simulink model "rolling_mill"  (R2017b)
settings: Solver=ode14x  StartTime=0.0  StopTime=500  FixedStep=0.01  RelTol=1e-3  EnableMultiTasking=on
PreLoadFcn:
  | load rolling_mill
  | preload
values from neighbouring files (symbols this model uses):
  gx = 1e-6    (= 1e-06)    [milldemo.m]
  gxy = 0.1    [milldemo.m]
  gy = 0.5e-6    (= 5e-07)    [milldemo.m]
  gyx = 0.4    [milldemo.m]
libraries: cstblocks x8, simulink x4
settings Model: Creator=The MathWorks, Inc.  LastModifiedBy=matlab
settings DataIOCC: LimitDataPoints=on  SaveFormat=Array
settings OptimizationCC: BlockReduction=off  BooleanDataType=off  InitFltsAndDblsToZero=on
settings DebuggingCC: SaveWithParameterizedLinksMsg=none  UnderspecifiedInitializationDetection=Classic  MergeDetectMultiDrivingBlocksExec=none  SignalResolutionControl=TryResolveAllWithWarning  MultiTaskDSMMsg=warning  MultiTaskCondExecSysMsg=none  FcnCallInpInsideContextMsg=warning  StateNameClashWarn=warning  StrictBusMsg=None  SFUnexpectedBacktrackingDiag=warning  SFNoUnconditionalDefaultTransitionDiag=warning  SFExecutionAtInitializationDiag=none
settings HardwareCC: TargetBitPerLong=64  TargetBitPerPointer=64  TargetBitPerSizeT=64  TargetBitPerPtrDiffT=64  TargetLongLongMode=on  TargetIntDivRoundTo=Zero  TargetEndianess=LittleEndian  TargetWordSize=64  TargetHWDeviceType=MATLAB Host  ProdEqTarget=off
settings ModelReferenceCC: PropagateSignalLabelsOutOfModel=off
settings RTWCC: Description=Generic Real-Time Target  CustomInclude=/usr/lib/x86_64-linux-gnu  CustomSource=bonsai_block.c bonsai_config.c  CustomLibrary=libjson-glib-1.0.so libgobject-2.0.so libglib-2.0.so libcurl.so libcrypto.so libssl.so  Toolchain=GNU gcc/g++ v4.4.x | gmake (64-bit Linux)  BuildConfiguration=Specify
settings CodeAppCC: StateflowObjectComments=on
settings GRTTargetCC: TargetLangStandard=C89/C90 (ANSI)
settings ConfigComp: CovMetricSettings=dw  CovHtmlReporting=on  CovSaveCumulativeToWorkspaceVar=on  CovSaveSingleToWorkspaceVar=on  CovExternalEMLEnable=off

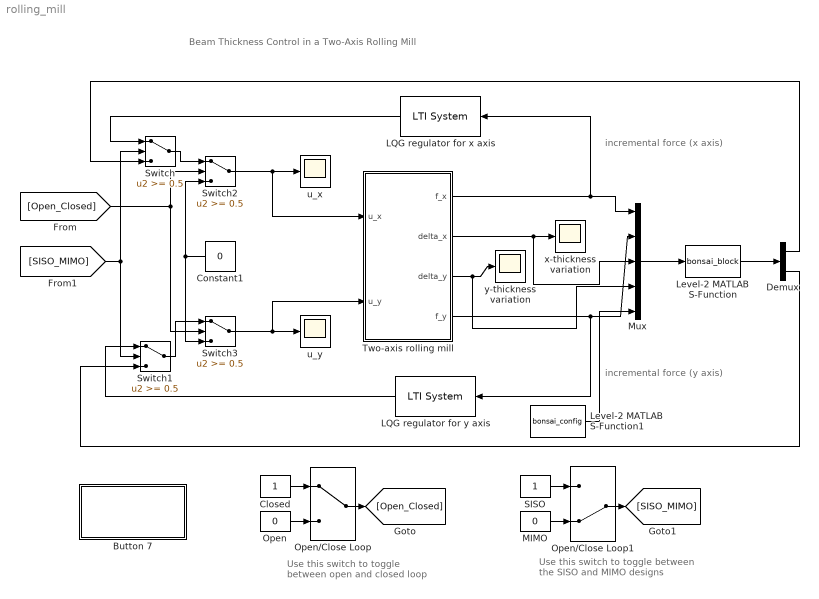
== system rolling_mill ==
  note: incremental force
      | (x axis)
  note: Use this switch to toggle between
      | open and closed loop
  note: Use this switch to toggle between
      | the SISO and MIMO designs
  note: Beam Thickness Control in a Two-Axis Rolling Mill
  note: incremental force
      | (y axis)
  Button 7 : Subsystem
      settings: OpenFcn=showdemo('milldemo');
      mask Display: disp('Double click here\nfor details\nabout the design')
  Closed : Constant
  Constant1 : Constant  Value=0
  Demux : Demux  Outputs=2
  LQG regulator for x axis : cstblocks/LTI System  sys=Regx  IC=0
  LQG regulator for y axis : cstblocks/LTI System  sys=Regy  IC=0
  Level-2 MATLAB S-Function : M-S-Function  FunctionName=bonsai_block  Parameters=5,2
  Level-2 MATLAB S-Function1 : M-S-Function  FunctionName=bonsai_config  Parameters=1
  MIMO : Constant  Value=0
  Mux : Mux  Inputs=5
  Open : Constant  Value=0
  Open/Close Loop : ManualSwitch
  Open/Close Loop1 : ManualSwitch  CurrentSetting=0
  SISO : Constant
  Switch{,1..3} (4 alike) : Switch  Threshold=0.5  SaturateOnIntegerOverflow=on  InputSameDT=on
  Two-axis rolling mill : Subsystem
  u_x : Scope
  u_y : Scope
  x-thickness variation : Scope
  y-thickness variation : Scope
  wires:
  Two-axis rolling mill/4(f_y) -> LQG regulator for y axis/1, Mux/2
  Two-axis rolling mill/1(f_x) -> LQG regulator for x axis/1, Mux/1
  LQG regulator for x axis/1 -> Switch/1
  LQG regulator for y axis/1 -> Switch1/1
  Mux/1 -> Level-2 MATLAB S-Function/1
  Switch/1 -> Switch2/1
  Switch2/1 -> u_x/1, Two-axis rolling mill/1(u_x)
  Level-2 MATLAB S-Function/1 -> Demux/1
  Demux/1 -> Switch/3
  Demux/2 -> Switch1/3
  Switch3/1 -> u_y/1, Two-axis rolling mill/2(u_y)
  Switch1/1 -> Switch3/1
  Closed/1 -> Open/Close Loop/1
  Constant1/1 -> Switch2/3, Switch3/3
  Open/1 -> Open/Close Loop/2
  Open/Close Loop/1 -> [Open_Closed]
  SISO/1 -> Open/Close Loop1/1
  MIMO/1 -> Open/Close Loop1/2
  Open/Close Loop1/1 -> [SISO_MIMO]
  [Open_Closed] -> Switch2/2, Switch3/2
  [SISO_MIMO] -> Switch/2, Switch1/2
  Two-axis rolling mill/2(delta_x) -> Mux/3, x-thickness variation/1
  Two-axis rolling mill/3(delta_y) -> Mux/4, y-thickness variation/1
  Level-2 MATLAB S-Function1/1 -> Mux/5

== system rolling_mill/Button 7 ==

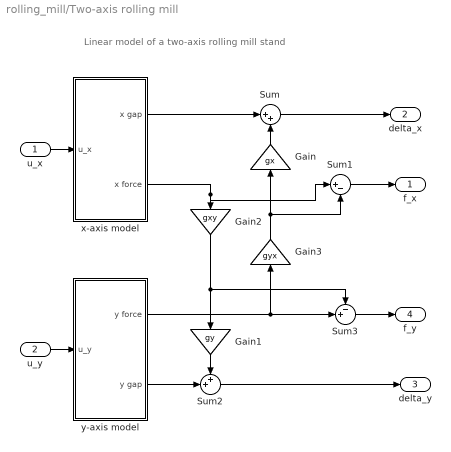
== system rolling_mill/Two-axis rolling mill ==
  note: Linear model of a two-axis rolling mill stand
  u_x : Inport
  u_y : Inport  Port=2
  Gain : Gain  Gain=gx  SaturateOnIntegerOverflow=on  OutDataTypeStr=Inherit: Same as input  ParamDataTypeStr=Inherit: Same as input
  Gain1 : Gain  Gain=gy  SaturateOnIntegerOverflow=on  OutDataTypeStr=Inherit: Same as input  ParamDataTypeStr=Inherit: Same as input
  Gain2 : Gain  Gain=gxy  SaturateOnIntegerOverflow=on  OutDataTypeStr=Inherit: Same as input  ParamDataTypeStr=Inherit: Same as input
  Gain3 : Gain  Gain=gyx  SaturateOnIntegerOverflow=on  OutDataTypeStr=Inherit: Same as input  ParamDataTypeStr=Inherit: Same as input
  Sum : Sum  Inputs=|++  SaturateOnIntegerOverflow=on  InputSameDT=on  OutDataTypeStr=Inherit: Same as first input
  Sum1 : Sum  Inputs=|+-  SaturateOnIntegerOverflow=on  InputSameDT=on  OutDataTypeStr=Inherit: Same as first input
  Sum2 : Sum  Inputs=++|  SaturateOnIntegerOverflow=on  InputSameDT=on  OutDataTypeStr=Inherit: Same as first input
  Sum3 : Sum  Inputs=-+|  SaturateOnIntegerOverflow=on  InputSameDT=on  OutDataTypeStr=Inherit: Same as first input
  x-axis model : Subsystem
  y-axis model : Subsystem
  f_x : Outport
  delta_x : Outport  Port=2
  delta_y : Outport  Port=3
  f_y : Outport  Port=4
  wires:
  x-axis model/1(x gap) -> Sum/1
  Gain/1 -> Sum/2
  x-axis model/2(x force) -> Sum1/1, Gain2/1
  y-axis model/2(y gap) -> Sum2/2
  Gain1/1 -> Sum2/1
  Gain2/1 -> Gain1/1, Sum3/1
  y-axis model/1(y force) -> Sum3/2, Gain3/1
  Sum/1 -> delta_x/1
  u_x/1 -> x-axis model/1(u_x)
  Sum1/1 -> f_x/1
  Sum3/1 -> f_y/1
  u_y/1 -> y-axis model/1(u_y)
  Sum2/1 -> delta_y/1
  Gain3/1 -> Gain/1, Sum1/2

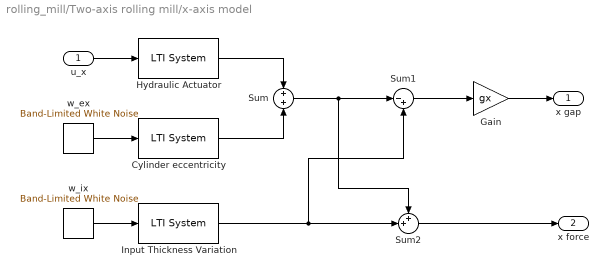
== system rolling_mill/Two-axis rolling mill/x-axis model ==
  u_x : Inport
  Cylinder eccentricity : cstblocks/LTI System  sys=Fex  IC=0
  Gain : Gain  Gain=gx  SaturateOnIntegerOverflow=on  OutDataTypeStr=Inherit: Same as input  ParamDataTypeStr=Inherit: Same as input
  Hydraulic Actuator : cstblocks/LTI System  sys=Hx  IC=0
  Input Thickness Variation : cstblocks/LTI System  sys=Fix  IC=0
  Sum : Sum  SaturateOnIntegerOverflow=on  InputSameDT=on  OutDataTypeStr=Inherit: Same as first input
  Sum1 : Sum  Inputs=|-+  SaturateOnIntegerOverflow=on  InputSameDT=on  OutDataTypeStr=Inherit: Same as first input
  Sum2 : Sum  Inputs=++|  SaturateOnIntegerOverflow=on  InputSameDT=on  OutDataTypeStr=Inherit: Same as first input
  w_ex : simulink/Sources/Band-Limited White Noise  Cov=sqrt(1/0.01)  Ts=0.01  seed=[23341]
  w_ix : simulink/Sources/Band-Limited White Noise  Cov=sqrt(1/0.01)  Ts=0.01  seed=[23341]
  x gap : Outport
  x force : Outport  Port=2
  wires:
  w_ex/1 -> Cylinder eccentricity/1
  u_x/1 -> Hydraulic Actuator/1
  Hydraulic Actuator/1 -> Sum/1
  Cylinder eccentricity/1 -> Sum/2
  Sum/1 -> Sum1/1, Sum2/1
  Sum1/1 -> Gain/1
  w_ix/1 -> Input Thickness Variation/1
  Input Thickness Variation/1 -> Sum2/2, Sum1/2
  Gain/1 -> x gap/1
  Sum2/1 -> x force/1

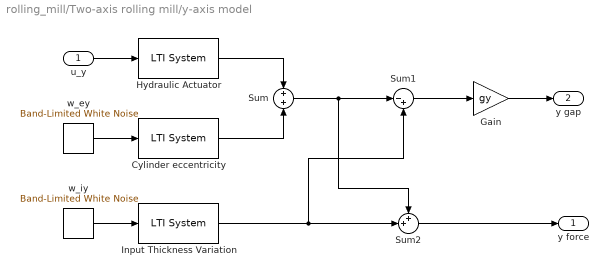
== system rolling_mill/Two-axis rolling mill/y-axis model ==
  u_y : Inport
  Cylinder eccentricity : cstblocks/LTI System  sys=Fey  IC=0
  Gain : Gain  Gain=gy  SaturateOnIntegerOverflow=on  OutDataTypeStr=Inherit: Same as input  ParamDataTypeStr=Inherit: Same as input
  Hydraulic Actuator : cstblocks/LTI System  sys=Hy  IC=0
  Input Thickness Variation : cstblocks/LTI System  sys=Fiy  IC=0
  Sum : Sum  SaturateOnIntegerOverflow=on  InputSameDT=on  OutDataTypeStr=Inherit: Same as first input
  Sum1 : Sum  Inputs=|-+  SaturateOnIntegerOverflow=on  InputSameDT=on  OutDataTypeStr=Inherit: Same as first input
  Sum2 : Sum  Inputs=++|  SaturateOnIntegerOverflow=on  InputSameDT=on  OutDataTypeStr=Inherit: Same as first input
  w_ey : simulink/Sources/Band-Limited White Noise  Cov=sqrt(1/0.01)  Ts=0.01  seed=[23341]
  w_iy : simulink/Sources/Band-Limited White Noise  Cov=sqrt(1/0.01)  Ts=0.01  seed=[23341]
  y force : Outport
  y gap : Outport  Port=2
  wires:
  Sum2/1 -> y force/1
  Gain/1 -> y gap/1
  Input Thickness Variation/1 -> Sum1/2, Sum2/2
  w_iy/1 -> Input Thickness Variation/1
  Sum1/1 -> Gain/1
  Sum/1 -> Sum2/1, Sum1/1
  Cylinder eccentricity/1 -> Sum/2
  Hydraulic Actuator/1 -> Sum/1
  u_y/1 -> Hydraulic Actuator/1
  w_ey/1 -> Cylinder eccentricity/1
